simulink model "low_pass"  (R2024b)
settings: Solver=VariableStepAuto  StartTime=0.0  StopTime=10.0  RelTol=1e-3
libraries: dspsrcs4 x1
settings Model: Creator=woutlyen  LastModifiedBy=woutlyen

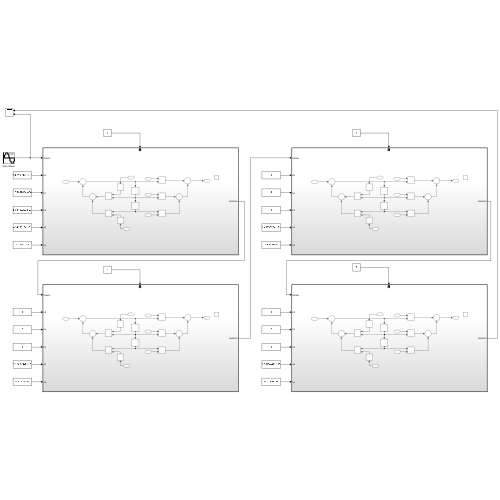
[thumbnail: Simulink's stored preview of the top-level diagram]
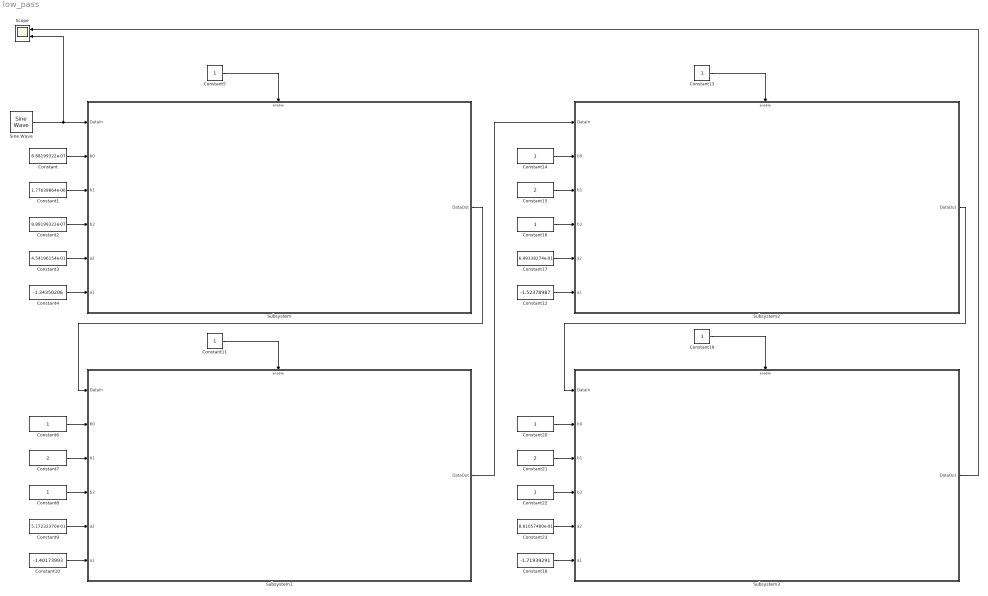
== system low_pass ==
  Constant : Constant  Value=8.88199322e-07  OutDataTypeStr=fixdt(1,27,23)
  Constant1 : Constant  Value=1.77639864e-06  OutDataTypeStr=fixdt(1,27,23)
  Constant10 : Constant  Value=-1.40173993  OutDataTypeStr=fixdt(1,27,23)
  Constant{5,11,13,19} (4 alike) : Constant  OutDataTypeStr=boolean
  Constant12 : Constant  Value=-1.52378987  OutDataTypeStr=fixdt(1,27,23)
  Constant{6,8,14,16,20,22} (6 alike) : Constant  OutDataTypeStr=fixdt(1,27,23)
  Constant15 : Constant  Value=2  OutDataTypeStr=fixdt(1,27,23)
  Constant17 : Constant  Value=6.49338274e-01  OutDataTypeStr=fixdt(1,27,23)
  Constant18 : Constant  Value=-1.71939291  OutDataTypeStr=fixdt(1,27,23)
  Constant2 : Constant  Value=8.88199322e-07  OutDataTypeStr=fixdt(1,27,23)
  Constant21 : Constant  Value=2  OutDataTypeStr=fixdt(1,27,23)
  Constant23 : Constant  Value=8.61057480e-01  OutDataTypeStr=fixdt(1,27,23)
  Constant3 : Constant  Value=4.54196154e-01  OutDataTypeStr=fixdt(1,27,23)
  Constant4 : Constant  Value=-1.34350206  OutDataTypeStr=fixdt(1,27,23)
  Constant7 : Constant  Value=2  OutDataTypeStr=fixdt(1,27,23)
  Constant9 : Constant  Value=5.17232370e-01  OutDataTypeStr=fixdt(1,27,23)
  Scope : Scope  NumInputPorts=2
  Sine Wave : dspsrcs4/Sine Wave  Amplitude=0.6  Frequency=2400  Phase=0  SampleMode=Discrete  OutComplex=Real  CompMethod=Table lookup  TableSize=Speed  SampleTime=1/48000  SamplesPerFrame=1  ResetState=Restart at time zero  OutputFrames=off  dataType=Fixed-point  wordLen=24  udDataType=sfix(16)  fracBitsMode=User-defined  numFracBits=23  OutDataTypeStr=fixdt(1,24,23)  LastOutDataTypeStr=fixdt(1,24,23)
  Subsystem : Subsystem
  Subsystem1 : Subsystem
  Subsystem2 : Subsystem
  Subsystem3 : Subsystem
  wires:
  Constant/1 -> Subsystem/2(b0)
  Constant1/1 -> Subsystem/3(b1)
  Constant2/1 -> Subsystem/4(b2)
  Constant3/1 -> Subsystem/5(a2)
  Constant4/1 -> Subsystem/6(a1)
  Constant5/1 -> Subsystem/Enable
  Constant10/1 -> Subsystem1/6(a1)
  Constant9/1 -> Subsystem1/5(a2)
  Constant7/1 -> Subsystem1/3(b1)
  Constant8/1 -> Subsystem1/4(b2)
  Constant6/1 -> Subsystem1/2(b0)
  Constant11/1 -> Subsystem1/Enable
  Constant15/1 -> Subsystem2/3(b1)
  Constant16/1 -> Subsystem2/4(b2)
  Constant14/1 -> Subsystem2/2(b0)
  Constant13/1 -> Subsystem2/Enable
  Constant12/1 -> Subsystem2/6(a1)
  Constant17/1 -> Subsystem2/5(a2)
  Constant21/1 -> Subsystem3/3(b1)
  Constant22/1 -> Subsystem3/4(b2)
  Constant18/1 -> Subsystem3/6(a1)
  Constant20/1 -> Subsystem3/2(b0)
  Constant19/1 -> Subsystem3/Enable
  Constant23/1 -> Subsystem3/5(a2)
  Subsystem/1(DataOut) -> Subsystem1/1(DataIn)
  Subsystem1/1(DataOut) -> Subsystem2/1(DataIn)
  Subsystem2/1(DataOut) -> Subsystem3/1(DataIn)
  Sine Wave/1 -> Subsystem/1(DataIn), Scope/2
  Subsystem3/1(DataOut) -> Scope/1

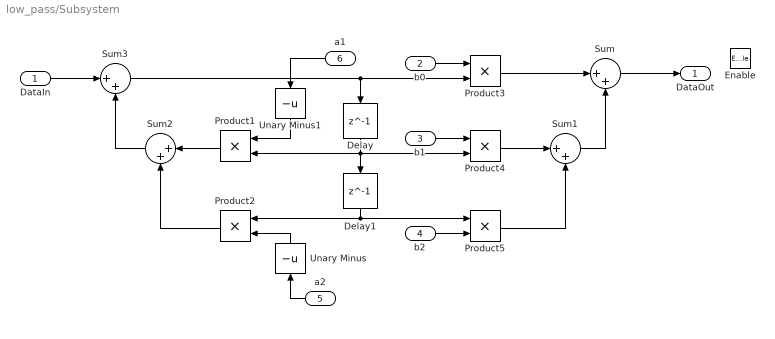
== system low_pass/Subsystem ==
  DataIn : Inport
  b0 : Inport  Port=2
  b1 : Inport  Port=3
  b2 : Inport  Port=4
  a2 : Inport  Port=5
  a1 : Inport  Port=6
  Enable : EnablePort
  Delay : Delay  DelayLength=1  InitialCondition=0
  Delay1 : Delay  DelayLength=1  InitialCondition=0
  Product{1..5} (5 alike) : Product  OutDataTypeStr=fixdt(1,27,23)
  Sum{,1..3} (4 alike) : Sum  Inputs=|++
  Unary Minus : UnaryMinus
  Unary Minus1 : UnaryMinus
  DataOut : Outport  VectorParamsAs1DForOutWhenUnconnected=off
  wires:
  Product4/1 -> Sum1/1
  b1/1 -> Product4/1
  Sum/1 -> DataOut/1
  Sum1/1 -> Sum/2
  b2/1 -> Product5/2
  a2/1 -> Unary Minus/1
  Delay1/1 -> Product2/1, Product5/1
  DataIn/1 -> Sum3/1
  Product2/1 -> Sum2/2
  Sum3/1 -> Delay/1, Product3/2
  Product1/1 -> Sum2/1
  Unary Minus1/1 -> Product1/1
  Sum2/1 -> Sum3/2
  Delay/1 -> Product4/2, Product1/2, Delay1/1
  Product3/1 -> Sum/1
  Unary Minus/1 -> Product2/2
  b0/1 -> Product3/1
  Product5/1 -> Sum1/2
  a1/1 -> Unary Minus1/1

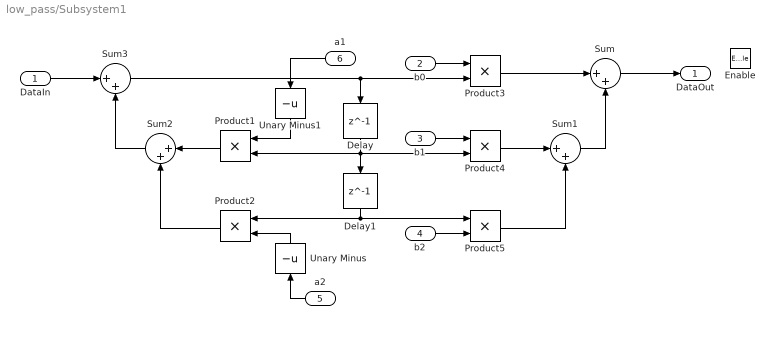
== system low_pass/Subsystem1 ==
  DataIn : Inport
  b0 : Inport  Port=2
  b1 : Inport  Port=3
  b2 : Inport  Port=4
  a2 : Inport  Port=5
  a1 : Inport  Port=6
  Enable : EnablePort
  Delay : Delay  DelayLength=1  InitialCondition=0
  Delay1 : Delay  DelayLength=1  InitialCondition=0
  Product{1..5} (5 alike) : Product  OutDataTypeStr=fixdt(1,27,23)
  Sum{,1..3} (4 alike) : Sum  Inputs=|++
  Unary Minus : UnaryMinus
  Unary Minus1 : UnaryMinus
  DataOut : Outport  VectorParamsAs1DForOutWhenUnconnected=off
  wires:
  Product4/1 -> Sum1/1
  b1/1 -> Product4/1
  Sum/1 -> DataOut/1
  Sum1/1 -> Sum/2
  b2/1 -> Product5/2
  a2/1 -> Unary Minus/1
  Delay1/1 -> Product2/1, Product5/1
  DataIn/1 -> Sum3/1
  Product2/1 -> Sum2/2
  Sum3/1 -> Delay/1, Product3/2
  Product1/1 -> Sum2/1
  Unary Minus1/1 -> Product1/1
  Sum2/1 -> Sum3/2
  Delay/1 -> Product4/2, Product1/2, Delay1/1
  Product3/1 -> Sum/1
  Unary Minus/1 -> Product2/2
  b0/1 -> Product3/1
  Product5/1 -> Sum1/2
  a1/1 -> Unary Minus1/1

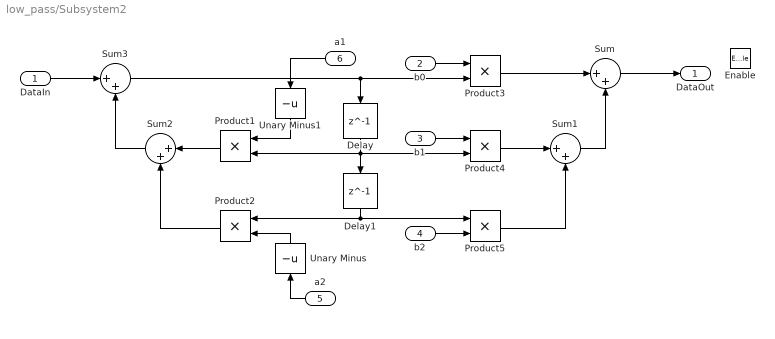
== system low_pass/Subsystem2 ==
  DataIn : Inport
  b0 : Inport  Port=2
  b1 : Inport  Port=3
  b2 : Inport  Port=4
  a2 : Inport  Port=5
  a1 : Inport  Port=6
  Enable : EnablePort
  Delay : Delay  DelayLength=1  InitialCondition=0
  Delay1 : Delay  DelayLength=1  InitialCondition=0
  Product{1..5} (5 alike) : Product  OutDataTypeStr=fixdt(1,27,23)
  Sum{,1..3} (4 alike) : Sum  Inputs=|++
  Unary Minus : UnaryMinus
  Unary Minus1 : UnaryMinus
  DataOut : Outport  VectorParamsAs1DForOutWhenUnconnected=off
  wires:
  Product4/1 -> Sum1/1
  b1/1 -> Product4/1
  Sum/1 -> DataOut/1
  Sum1/1 -> Sum/2
  b2/1 -> Product5/2
  a2/1 -> Unary Minus/1
  Delay1/1 -> Product2/1, Product5/1
  DataIn/1 -> Sum3/1
  Product2/1 -> Sum2/2
  Sum3/1 -> Delay/1, Product3/2
  Product1/1 -> Sum2/1
  Unary Minus1/1 -> Product1/1
  Sum2/1 -> Sum3/2
  Delay/1 -> Product4/2, Product1/2, Delay1/1
  Product3/1 -> Sum/1
  Unary Minus/1 -> Product2/2
  b0/1 -> Product3/1
  Product5/1 -> Sum1/2
  a1/1 -> Unary Minus1/1

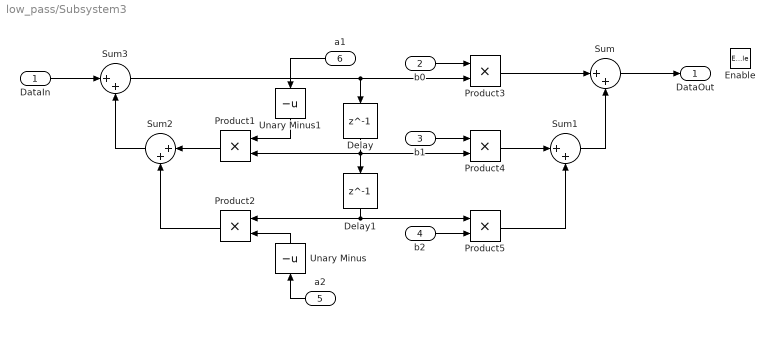
== system low_pass/Subsystem3 ==
  DataIn : Inport
  b0 : Inport  Port=2
  b1 : Inport  Port=3
  b2 : Inport  Port=4
  a2 : Inport  Port=5
  a1 : Inport  Port=6
  Enable : EnablePort
  Delay : Delay  DelayLength=1  InitialCondition=0
  Delay1 : Delay  DelayLength=1  InitialCondition=0
  Product{1..5} (5 alike) : Product  OutDataTypeStr=fixdt(1,27,23)
  Sum{,1..3} (4 alike) : Sum  Inputs=|++
  Unary Minus : UnaryMinus
  Unary Minus1 : UnaryMinus
  DataOut : Outport  VectorParamsAs1DForOutWhenUnconnected=off
  wires:
  Product4/1 -> Sum1/1
  b1/1 -> Product4/1
  Sum/1 -> DataOut/1
  Sum1/1 -> Sum/2
  b2/1 -> Product5/2
  a2/1 -> Unary Minus/1
  Delay1/1 -> Product2/1, Product5/1
  DataIn/1 -> Sum3/1
  Product2/1 -> Sum2/2
  Sum3/1 -> Delay/1, Product3/2
  Product1/1 -> Sum2/1
  Unary Minus1/1 -> Product1/1
  Sum2/1 -> Sum3/2
  Delay/1 -> Product4/2, Product1/2, Delay1/1
  Product3/1 -> Sum/1
  Unary Minus/1 -> Product2/2
  b0/1 -> Product3/1
  Product5/1 -> Sum1/2
  a1/1 -> Unary Minus1/1
